simulink model "ctsdm_3stage_bk"  (R2021a)
settings: Solver=VariableStepAuto  StartTime=0.0  StopTime=time  RelTol=1e-3
undefined symbols (not defined in the file or in its folder): c1, c2, c3, fin, fs, k1, k2, k3, n, osr, Ts
libraries: SDtoolbox x1
settings Model: Creator=weihaoyu  LastModifiedBy=weihaoyu

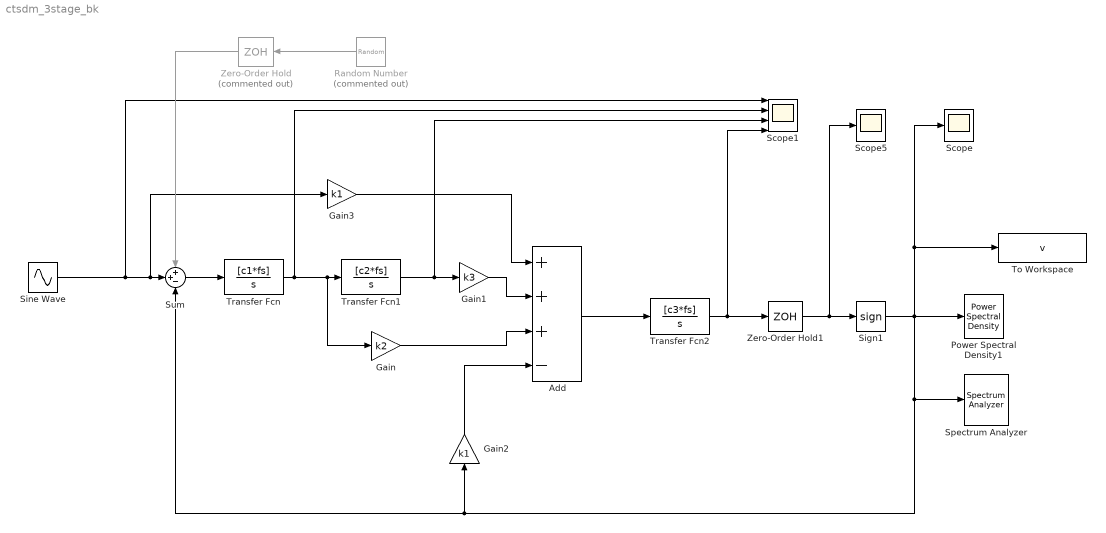
== system ctsdm_3stage_bk ==
  Add : Sum  Inputs=+++-
  Gain : Gain  Gain=k2
  Gain1 : Gain  Gain=k3
  Gain2 : Gain  Gain=k1
  Gain3 : Gain  Gain=k1
  Power Spectral Density1 : SDtoolbox/Power Spectral Density  SN=2  Fs=fs  fBL=0  fBH=fs/(2*osr)  Fin=fin  N=n  Ntransient=0  VW=off  savename=savemat  Scale_type=logarithmic
  Random Number : RandomNumber  Commented=on  Variance=6.91e-6  SampleTime=Ts
  Scope : Scope
  Scope1 : Scope  NumInputPorts=4
  Scope5 : Scope
  Sign1 : Signum
  Sine Wave : Sin  Amplitude=0.8  Frequency=fin*2*pi  SampleTime=0
  Spectrum Analyzer : SpectrumAnalyzer
  Sum : Sum  Inputs=++-
  To Workspace : ToWorkspace  VariableName=v  SampleTime=1/fs
  Transfer Fcn : TransferFcn  Numerator=[c1*fs]  Denominator=[1 0]
  Transfer Fcn1 : TransferFcn  Numerator=[c2*fs]  Denominator=[1 0]
  Transfer Fcn2 : TransferFcn  Numerator=[c3*fs]  Denominator=[1 0]
  Zero-Order Hold : ZeroOrderHold  Commented=on  SampleTime=-1
  Zero-Order Hold1 : ZeroOrderHold  SampleTime=1/fs
  wires:
  Transfer Fcn/1 -> Scope1/2, Gain/1, Transfer Fcn1/1
  Transfer Fcn1/1 -> Scope1/3, Gain1/1
  Gain1/1 -> Add/2
  Gain/1 -> Add/3
  Add/1 -> Transfer Fcn2/1
  Transfer Fcn2/1 -> Scope1/4, Zero-Order Hold1/1
  Sign1/1 -> Power Spectral Density1/1, Spectrum Analyzer/1, Sum/3, Gain2/1, To Workspace/1, Scope/1
  Gain2/1 -> Add/4
  Sine Wave/1 -> Scope1/1, Gain3/1, Sum/2
  Sum/1 -> Transfer Fcn/1
  Gain3/1 -> Add/1
  Zero-Order Hold1/1 -> Sign1/1, Scope5/1
  Random Number/1 -> Zero-Order Hold/1
  Zero-Order Hold/1 -> Sum/1
